simulink model "model_problem5"  (R2020a)
settings: Solver=VariableStepAuto  StartTime=0.0  StopTime=10.0  RelTol=1e-3
settings Model: Creator=Prateek  LastModifiedBy=Prateek

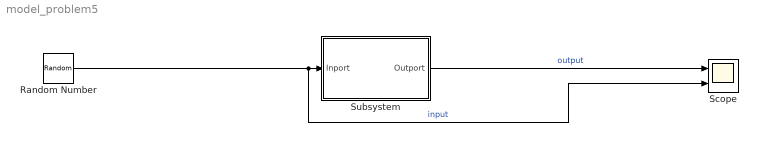
== system model_problem5 ==
  Random Number : RandomNumber  SampleTime=0.1
  Scope : Scope  NumInputPorts=2
  Subsystem : Subsystem
  wires:
  Subsystem/1(Outport) -> Scope/1  "output"
  Random Number/1 -> Scope/2, Subsystem/1(Inport)  "input"

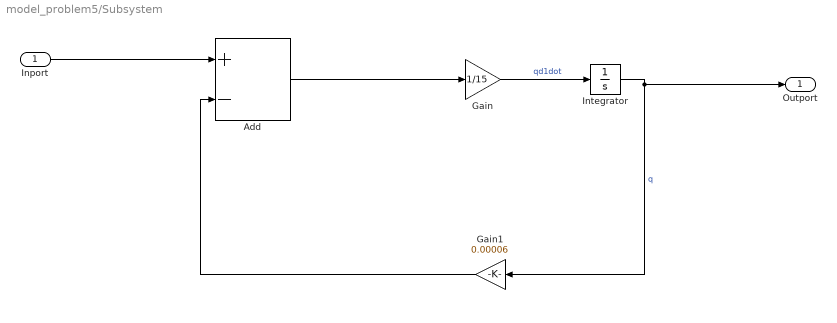
== system model_problem5/Subsystem ==
  Inport : Inport
  Add : Sum  Inputs=+-
  Gain : Gain  Gain=1/15
  Gain1 : Gain  Gain=0.00006
  Integrator : Integrator
  Outport : Outport
  wires:
  Integrator/1 -> Outport/1, Gain1/1  "q"
  Inport/1 -> Add/1
  Gain/1 -> Integrator/1  "qd1dot"
  Gain1/1 -> Add/2
  Add/1 -> Gain/1
